simulink model "s5_c0_uio"  (R2023a)
settings: Solver=FixedStepAuto  StartTime=0.0  StopTime=32  FixedStep=1E-3  RelTol=1e-3
undefined symbols (not defined in the file): A, B1, C, C_obs1, C_obs2, CI, E_obs1, E_obs2, L_obs1, L_obs2, N_obs1, N_obs2
settings Model: Creator=felipe  LastModifiedBy=felipe

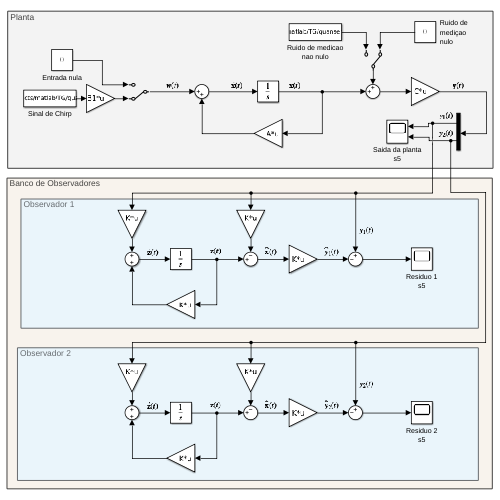
[thumbnail: Simulink's stored preview of the top-level diagram]
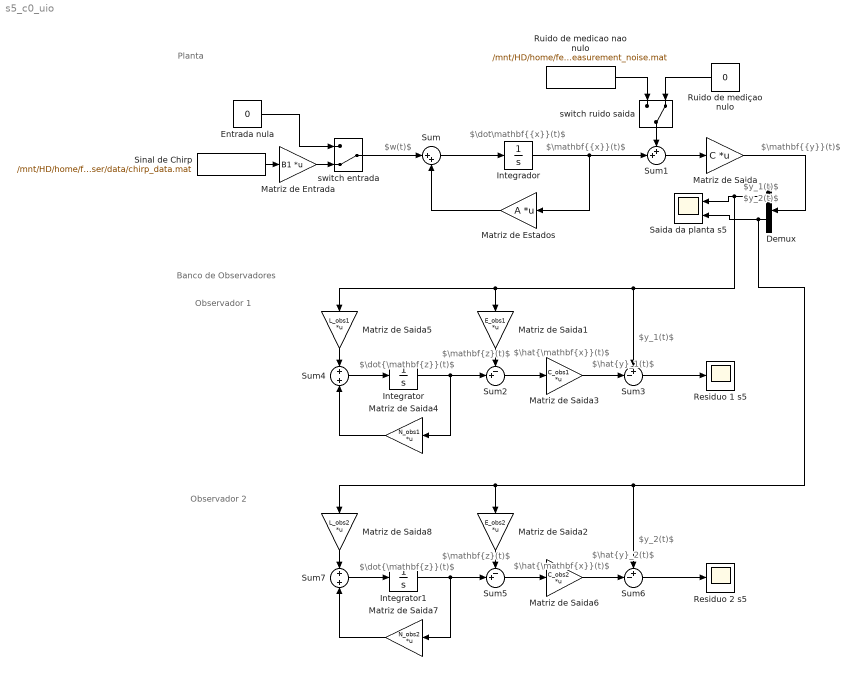
== system s5_c0_uio ==
  note: Banco de Observadores
  note: Observador 1
  note: $w(t)$
  note: Planta
  note: $\dot\mathbf{{x}}(t)$
  note: $\mathbf{{x}}(t)$
  note: $\mathbf{{y}}(t)$
  note: Observador 2
  note: $y_1(t)$
  note: $y_2(t)$
  note: $y_1(t)$
  note: $y_2(t)$
  note: $\mathbf{z}(t)$
  note: $\dot{\mathbf{z}}(t)$
  note: $\hat{\mathbf{x}}(t)$
  note: $\hat{y}_1(t)$
  note: $\hat{y}_2(t)$
  note: $\hat{\mathbf{x}}(t)$
  note: $\mathbf{z}(t)$
  note: $\dot{\mathbf{z}}(t)$
  Demux : Demux  Outputs=2
  Entrada nula : Constant  Value=0
  Integrador : Integrator  InitialCondition=CI
  Integrator : Integrator
  Integrator1 : Integrator
  Matriz de Entrada : Gain  Gain=B1  Multiplication=Matrix(K*u)
  Matriz de Estados : Gain  Gain=A  Multiplication=Matrix(K*u)
  Matriz de Saida : Gain  Gain=C  Multiplication=Matrix(K*u)
  Matriz de Saida1 : Gain  Gain=E_obs1  Multiplication=Matrix(K*u)
  Matriz de Saida2 : Gain  Gain=E_obs2  Multiplication=Matrix(K*u)
  Matriz de Saida3 : Gain  Gain=C_obs1  Multiplication=Matrix(K*u)
  Matriz de Saida4 : Gain  Gain=N_obs1  Multiplication=Matrix(K*u)
  Matriz de Saida5 : Gain  Gain=L_obs1  Multiplication=Matrix(K*u)
  Matriz de Saida6 : Gain  Gain=C_obs2  Multiplication=Matrix(K*u)
  Matriz de Saida7 : Gain  Gain=N_obs2  Multiplication=Matrix(K*u)
  Matriz de Saida8 : Gain  Gain=L_obs2  Multiplication=Matrix(K*u)
  Residuo 1 s5 : Scope
  Residuo 2 s5 : Scope
  Ruido de mediçao nulo : Constant  Value=0
  Ruido de medicao nao nulo : FromFile  FileName=/mnt/HD/home/felipe/Projects/matlab/TG/quanser/data/measurement_noise.mat  SampleTime=0
  Saida da planta s5 : Scope  NumInputPorts=2
  Sinal de Chirp : FromFile  FileName=/mnt/HD/home/felipe/Projects/matlab/TG/quanser/data/chirp_data.mat  SampleTime=0
  Sum : Sum  Inputs=|++
  Sum1 : Sum  Inputs=++|
  Sum2 : Sum  Inputs=-+|
  Sum3 : Sum  Inputs=+-|
  Sum4 : Sum
  Sum5 : Sum  Inputs=-+|
  Sum6 : Sum  Inputs=+-|
  Sum7 : Sum
  switch entrada : ManualSwitch  CurrentSetting=0
  switch ruido saida : ManualSwitch  CurrentSetting=0
  wires:
  Sum/1 -> Integrador/1
  Matriz de Estados/1 -> Sum/2
  Integrador/1 -> Sum1/2, Matriz de Estados/1
  Matriz de Saida/1 -> Demux/1
  Sinal de Chirp/1 -> Matriz de Entrada/1
  Matriz de Entrada/1 -> switch entrada/2
  Entrada nula/1 -> switch entrada/1
  Sum1/1 -> Matriz de Saida/1
  switch ruido saida/1 -> Sum1/1
  Ruido de mediçao nulo/1 -> switch ruido saida/2
  Ruido de medicao nao nulo/1 -> switch ruido saida/1
  switch entrada/1 -> Sum/1
  Sum3/1 -> Residuo 1 s5/1
  Demux/1 -> Sum3/1, Matriz de Saida1/1, Matriz de Saida5/1, Saida da planta s5/1
  Sum2/1 -> Matriz de Saida3/1
  Matriz de Saida1/1 -> Sum2/1
  Matriz de Saida3/1 -> Sum3/2
  Integrator/1 -> Sum2/2, Matriz de Saida4/1
  Matriz de Saida4/1 -> Sum4/2
  Matriz de Saida5/1 -> Sum4/1
  Sum4/1 -> Integrator/1
  Matriz de Saida7/1 -> Sum7/2
  Matriz de Saida6/1 -> Sum6/2
  Integrator1/1 -> Sum5/2, Matriz de Saida7/1
  Sum6/1 -> Residuo 2 s5/1
  Sum5/1 -> Matriz de Saida6/1
  Matriz de Saida2/1 -> Sum5/1
  Matriz de Saida8/1 -> Sum7/1
  Demux/2 -> Matriz de Saida8/1, Matriz de Saida2/1, Sum6/1, Saida da planta s5/2
  Sum7/1 -> Integrator1/1
